simulink model "main_RI_LIEKF"  (R2023a)
settings: Solver=FixedStepAuto  StartTime=0.0  StopTime=220  FixedStep=0.01  RelTol=1e-3
InitFcn:
  | initNavigation0612_AOA;
values from neighbouring files (symbols this model uses):
  CF_enable = 0    [initNavigation.m]
  dt = 0.01    [initNavigation.m]
  dtDelay = -0.03    [initNavigation.m]
  g0 = 9.795    [initNavigation.m]
  gam0_rad = 0/57.3    (= 0)    [initNavigation.m]
  H_sensor_type = 0    [initNavigation.m]
  KF_enable = 1    [initNavigation.m]
  P0 = diag([1*ones(3,1);0.01*ones(3,1);0.1*ones(3,1);0.001*ones(3,1);0.00001*ones(3,1)])    [initNavigation.m]
  P0_RIEKF = diag([1*ones(3,1);0.01*ones(3,1);0.1*ones(3,1);0.001*ones(3,1);0.00001*ones(3,1);      0.01*ones(3,1);[0;2;2]/57.3;[0.1;0.1;0.1]])^2    [initNavigation.m]
  pd0 = 0    [initNavigation.m]
  pe0 = 0    [initNavigation.m]
  phi0_rad = 0/57.3    (= 0)    [initNavigation.m]
  pn0 = 0    [initNavigation.m]
  psi = -178    [initNavigation.m]
  psi0_rad = 0/57.3    (= 0)    [initNavigation.m]
  state_dim = 24    [initNavigation.m]
  Time = 0:0.01:(size(traindata.AttackAngle,1) - 1)*0.01    [NNLiftCoefficientFit.m]
  vd0 = 0    [initNavigation.m]
  ve0 = 0    [initNavigation.m]
  vn0 = 0    [initNavigation.m]
undefined symbols (not defined in the file or in its folder): DiscIntNeverNeededParam, Discrete, INS_CONST, INS_EXPORT, INS_PARAM, magnitude, p, param, pInitialization, sys
libraries: simulink x69, simulink_extras x64, dspstat3 x56, sharedtransform x49, ctrlSharedLib x36, sharedTrackingLibrary x17, FMT_Model_Lib x13, matrix_library x12, deeplib x4, dspsolvers x4, vrlib x4, aerolibconvert2 x1
(part 22 of 22)

== matlab function main_RI_LIEKF/State estimation/bak1/Error State Kalman Filter/Simulink Function - GPS Measurements1/MATLAB Function1 ==
  data: H output; Cbn input; dt input
function H = calH(Cbn, dt)
    

    H = zeros(3,18);
    % 

    H(1:3,4:6) = eye(3);
    H(1:3,16:18) = -Cbn * dt;
end

== matlab function main_RI_LIEKF/State estimation/bak1/Error State Kalman Filter/Simulink Function - State Transition/Cal Phi/MATLAB Function1 ==
  data: vn input; Phi output; pn input; Rbn input; dt input
function Phi = fcn(vn,pn, Rbn,dt)
    
    %{
    F.block(0, 0, 3, 3) = exp_so3(-w_hat * dt);
        F.block(0, 9, 3, 3).noalias() = -exp_so3(-w_hat * dt) * Jr_so3(-w_hat * dt) * dt;
        F.block(9, 9, 3, 3).setIdentity();
        F.block(6, 0, 3, 3).noalias() = -R_Gtoi.transpose() * skew_x(a_hat * dt);
        F.block(6, 6, 3, 3).setIdentity();
        F.block(6, 12, 3, 3) = -R_Gtoi.transpose() * dt;
        F.block(12, 12, 3, 3).setIdentity();
        F.block(3, 0, 3, 3).noalias() = -0.5 * R_Gtoi.transpose() * skew_x(a_hat * dt * dt);
        F.block(3, 6, 3, 3) = Eigen::Matrix3d::Identity() * dt;
        F.block(3, 12, 3, 3) = -0.5 * R_Gtoi.transpose() * dt * dt;
        F.block(3, 3, 3, 3).setIdentity();
        Eigen::Matrix<double, 15, 12> G = Eigen::Matrix<double, 15, 12>::Zero();
    %}
    %
    %
    %F = [0_33         0_33  0_33   -Rbn          0_33]
    %    [skew(gn)     0_33  0_33  -skew(vn)Rbn   -Rbn]
    %    [0.5*skew(gn) I_33  0_33  -skew(pn)Rbn   -Rbn]
    %    [         0_69                  I66          ]
    Phi = zeros(15,15);
    g0 = 9.79;
    gn = [0;0;-g0];
    F  = zeros(15,15);
    F(1:3,10:12) = -Rbn;
    F(4:6,1:3)   = skewMat(gn);
    F(4:6,10:12) = -skewMat(vn)*Rbn;
    F(4:6,13:15) = -Rbn;
    F(7:9,4:6)   = eye(3);
    F(7:9,1:3)   = 0.5*skewMat(gn);
    F(7:9,10:12) = -skewMat(pn)*Rbn;
    F(7:9,13:15) = -Rbn;
    %F(10:15,10:15) = eye(6);
    Phi = eye(15) + F * dt;

end

== matlab function main_RI_LIEKF/State estimation/bak1/Error State Kalman Filter/Simulink Function - State Transition/MATLAB Function ==
  data: Rbn input; G output; vn input; pn input; dt input
function G = fcn(Rbn, vn,pn, dt)
    % G.block(0, 0, 3, 3) = -exp_so3(-w_hat * dt) * Jr_so3(-w_hat * dt) * dt;
    %    G.block(6, 3, 3, 3) = -R_Gtoi.transpose() * dt;
    %    G.block(3, 3, 3, 3) = -0.5 * R_Gtoi.transpose() * dt * dt;
    %    G.block(9, 6, 3, 3).setIdentity();
    %    G.block(12, 9, 3, 3).setIdentity();

    G = zeros(15,12);
    % G(1:3,1:3) = -  Rbn * dt;
    % G(4:6,1:3) = -skewMat(vn)*Rbn* dt;
    % G(4:6,4:6) =  - Rbn;
    % G(7:9,1:3) = -skewMat(pn)*Rbn * dt;
    % G(7:9,4:6) =  - Rbn;
    % G(10:12,7:9) = eye(3)*dt;
    % G(13:15,10:12) = eye(3)*dt;
    G(1:3,1:3) = -  Rbn;
    G(4:6,1:3) = -skewMat(vn)*Rbn;
    G(4:6,4:6) =  - Rbn;
    G(7:9,1:3) = -skewMat(pn)*Rbn;
    G(7:9,4:6) =  - Rbn;
    G(10:12,7:9) = eye(3);
    G(13:15,10:12) = eye(3);
    G = G*double(dt);
end

== matlab function main_RI_LIEKF/State estimation/15dim KF1/Error State Kalman Filter/Cal Phi/MATLAB Function1 ==
  data: axyz input; Phi output; Cnb input; wxyz input; dt input
function Phi = fcn(axyz, Cnb, wxyz,dt)
    
    %{
    F.block(0, 0, 3, 3) = exp_so3(-w_hat * dt);
        F.block(0, 9, 3, 3).noalias() = -exp_so3(-w_hat * dt) * Jr_so3(-w_hat * dt) * dt;
        F.block(9, 9, 3, 3).setIdentity();
        F.block(6, 0, 3, 3).noalias() = -R_Gtoi.transpose() * skew_x(a_hat * dt);
        F.block(6, 6, 3, 3).setIdentity();
        F.block(6, 12, 3, 3) = -R_Gtoi.transpose() * dt;
        F.block(12, 12, 3, 3).setIdentity();
        F.block(3, 0, 3, 3).noalias() = -0.5 * R_Gtoi.transpose() * skew_x(a_hat * dt * dt);
        F.block(3, 6, 3, 3) = Eigen::Matrix3d::Identity() * dt;
        F.block(3, 12, 3, 3) = -0.5 * R_Gtoi.transpose() * dt * dt;
        F.block(3, 3, 3, 3).setIdentity();
        Eigen::Matrix<double, 15, 12> G = Eigen::Matrix<double, 15, 12>::Zero();
    %}
    Phi = zeros(15,15);
    % 
    Phi(1:3,1:3) = eye(3);      %P-P
    Phi(1:3,4:6) = dt * eye(3); %P-V
    Phi(1:3,7:9) = -0.5*Cnb'*skewMat(axyz * dt * dt); %P-the
    % 
    Phi(4:6,4:6) = eye(3);
    Phi(4:6,7:9) = -Cnb' * skewMat(axyz * dt);
    Phi(4:6,10:12) = -Cnb'*dt ;
    % 
    Phi(7:9,7:9) = exp_so3(-wxyz * dt);     %the-the
    Phi(7:9,13:15) = -exp_so3(-wxyz * dt) * Jl_so3(wxyz * dt) * dt; %the-bias g
    % 
    Phi(10:12,10:12) = eye(3);
    % % 
    Phi(13:15,13:15) = eye(3);
    % 
    Phi(1:3,10:12) = - 0.5*Cnb' * dt * dt;

end

== matlab function main_RI_LIEKF/State estimation/ER EKF/INS propogation/Init_PVQ/Horizontal_attitude2/Hem2JPL1 ==
  data: q input; y output
function y = fcn(q)

y = [q(2:4);q(1)];

== matlab function main_RI_LIEKF/State estimation/ER EKF/INS propogation/Init_PVQ/Horizontal_attitude2/Hem2JPL2 ==
  data: q input; y output
function y = fcn(q)

y = [q(2:4);q(1)];

== matlab function main_RI_LIEKF/State estimation/RI EKF/INS propogation/AOA//SA//Vwind update/Subsystem/MATLAB Function3 ==
  data: axyz input; Cy output; TAS input; alpha input; beta input
function Cy = fcn(axyz, TAS,alpha,beta)
ax = axyz(1);
ay = axyz(2);
az = axyz(3);

mess = 6.9;
g = 9.79;
rou = 1.225;
a = 1.4;
b = 0.36;
S = a*b;

q = 0.5 * rou * TAS^2;
ays = -ax .* cos(alpha).*sin(beta) + ay .* cos(beta) - az .* sin(alpha).* sin(beta);
% azs = -ax * sin(alpha) + az * cos(alpha);
Cy = mess * ays / (q * S);
end

== matlab function main_RI_LIEKF/State estimation/RI EKF/INS propogation/AOA//SA//Vwind update/Subsystem/LSTM predict/MATLAB Function5 ==
  data: X input; X_nYPred output
function X_nYPred = LSTMnet(X)
    sig_X = [0.1167;0.1277;0.0579];
    sig_Y = 0.0451;
    mu_X = [0.0587;0.5185;-0.0515];
    mu_Y = 0.1011;
    X_norm = (X - mu_X) ./ sig_X;
    persistent X_nYPredorm_store;
    if isempty(X_nYPredorm_store)
        X_nYPredorm_store = zeros(1000,3);
    end

    X_nYPredorm_store = [X_nYPredorm_store(2:end,:);X_norm'];
    %[~,YPred_seq] = predictAndUpdateState(net.net,X_nYPredorm_store);
     X_nYPred = single(X_nYPredorm_store);
    % YPred_seq = predict(net.net,X_nYPredorm_store');
    % YPred_test = YPred_seq(end);
    % YPred_test = double(YPred_test* sig_Y + mu_Y)*57.3;

end

== matlab function main_RI_LIEKF/State estimation/ER EKF/Error State Kalman Filter/Simulink Function - State Transition/MATLAB Function ==
  data: Cnb input; G output; wxyz input; dt input
function G = fcn(Cnb, wxyz, dt)
    % G.block(0, 0, 3, 3) = -exp_so3(-w_hat * dt) * Jr_so3(-w_hat * dt) * dt;
    %    G.block(6, 3, 3, 3) = -R_Gtoi.transpose() * dt;
    %    G.block(3, 3, 3, 3) = -0.5 * R_Gtoi.transpose() * dt * dt;
    %    G.block(9, 6, 3, 3).setIdentity();
    %    G.block(12, 9, 3, 3).setIdentity();
    
    G = zeros(15,12);
    G(7:9,4:6) = -exp_so3(-wxyz * dt) * Jr_so3(- wxyz * dt) * dt;
    G(1:3,1:3) = -0.5 * Cnb' * dt * dt;
    G(4:6,1:3) = -Cnb' * dt;
    G(10:12,7:9) = eye(3);
    G(13:15,10:12) = eye(3);
    
%     G(16:18,13:15) = eye(3);
%     G(16:18,1:3) = -eye(3);
end

== matlab function main_RI_LIEKF/State estimation/RI EKF/INS propogation/AOA//SA//Vwind update/Subsystem/LSTM predict/MATLAB Function6 ==
  data: YPred_test input; YPred_test_out output
function YPred_test_out = LSTMnet(YPred_test)
    sig_X = [0.1167;0.1277;0.0579];
    sig_Y = 0.0451;
    mu_X = [0.0587;0.5185;-0.0515];
    mu_Y = 0.1011;
    YPred_test_out = YPred_test(end);
    YPred_test_out = single(YPred_test_out* sig_Y + mu_Y)*57.3;

end

== matlab function main_RI_LIEKF/State estimation/15dim KF1/Error State Kalman Filter/Cal Q/MATLAB Function1 ==
  data: Qd output; Cnb input; wxyz input; dt input
function Qd = fcn(Cnb, wxyz, dt)
    % G.block(0, 0, 3, 3) = -exp_so3(-w_hat * dt) * Jr_so3(-w_hat * dt) * dt;
    %    G.block(6, 3, 3, 3) = -R_Gtoi.transpose() * dt;
    %    G.block(3, 3, 3, 3) = -0.5 * R_Gtoi.transpose() * dt * dt;
    %    G.block(9, 6, 3, 3).setIdentity();
    %    G.block(12, 9, 3, 3).setIdentity();
    
    G = zeros(15,12);
    G(7:9,4:6) = -exp_so3(-wxyz * dt) * Jl_so3(wxyz * dt) * dt;
    G(1:3,1:3) = -0.5 * Cnb' * dt * dt;
    G(4:6,1:3) = -Cnb' * dt;
    G(10:12,7:9) = eye(3);
    G(13:15,10:12) = eye(3);
     
    Q = zeros(12,12);
%     noises_sigma_a_2 = 2.0000e-4^2;
%     noises_sigma_w_2 = 1.6968e-4^2;
%     noises_sigma_ab_2 = 3.0000e-4^2;
%     noises_sigma_wb_2 = 1.9393e-5^2;
    noises_sigma_a_2 = 0.0001^2;
    noises_sigma_w_2 = 0.0025^2;
    noises_sigma_ab_2 = 3.0000e-5^2;
    noises_sigma_wb_2 = 0.0002^2;
    Q = diag([noises_sigma_a_2 / dt * ones(3,1); ...
                noises_sigma_w_2 / dt * ones(3,1); ...
                noises_sigma_ab_2 * dt * ones(3,1); ...
                noises_sigma_wb_2 * dt * ones(3,1);]);
    
    Qd = zeros(15,15);
    Qd = G * Q * G';
    Qd = 0.5 * (Qd + Qd');
end

== matlab function main_RI_LIEKF/State estimation/15dim KF1/Error State Kalman Filter/GNSS//INS Kalman Filter1/CalculatePL/Discrete-Time KF - Calculate PLMZ ==
  settings: updateMethod=DISCRETE  sampleTime=pInitialization.Ts
  data: A input; L output; M output; Z output; C input; Q input; R input; N input; P input; PNew output; isEnabled input
function [L,M,Z,PNew] = ctrlKalmanFilterDTCalculatePL_0115(A,C,Q,R,N,P,isEnabled)
% ctrlKalmanFilterDTCalculatePL Calculate the Kalman gain L for current
% time step and P for the next time step (PNew) for discrete-time Kalman
% filtering with time-varying system matrices.
%
%   Inputs:
%     A, C, Q, R, N, P - System and noise covariance matrices. See kalman()
%     isEnabled        - Is measurement update being done at this time
%                        step?
%
%   Outputs:
%      L    - Kalman gain to get x[k+1|k] from x[k|k-1] and y[k]
%      M    - Kalman gain to get x[k|k] from x[k|k-1] and y[k]
%      Z    - State estimation covariance of x[k|k]
%      PNew - P[k+1], state estimation error covariance for the next time
%             step

%   Copyright 2014-2019 The MathWorks, Inc.

%#codegen
if isEnabled
    % Do measurement update
    yCov = C*P*C.'+R;
    L = (A*P*C.'+N) / yCov;
    M = P*C.' / yCov;
    
    Abar = eye(size(A,1),'like', A) - M*C;
    Z = Abar*P*Abar.' + M*R*M.';
    
    NRinv = N/R;
    Abar = A - NRinv*C;
    PNew = Abar*Z*Abar.' + Q - NRinv*N.';
else
    % No measurement update
    L = zeros(size(A,1),size(C,1),'like',A);
    M = L;
    Z = P;
    PNew = A*P*A.' + Q;
end
end

== matlab function main_RI_LIEKF/State estimation/0609bk/Error State Kalman Filter/Extended Kalman Filter1/Correct1/IGG_check/MATLAB Function ==
  data: err input; w output; k0 input; k1 input; zk0 input; zk1 input
function w = fcn(err,k0,k1,zk0,zk1)
    err = abs(err);  w = err;
    for k=1:2
        if err(k)<=k0,    w(k)=1;
        elseif err(k)>k1, w(k)=0;
        else,             w(k)=k0/err(k);  
        end
    end
        if err(3)<=zk0,    w(3)=1;
        elseif err(3)>zk1, w(3)=0;
        else,             w(3)=zk0/err(3);  
        end
end

== matlab function main_RI_LIEKF/State estimation/15dim KF1/Error State Kalman Filter/GNSS//INS Kalman Filter1/CovarianceOutputConfigurator/decideOutput/SqrtUsedFcn ==
  data: u input; P output; isSqrtUsed input
function P = outputCovariance(u,isSqrtUsed)
   
   % Determine if the Square-Root algorithm was used
   if isSqrtUsed
      P = u*u.';
   else
      P = u;
   end   
end

== matlab function main_RI_LIEKF/State estimation/15dim KF1/Error State Kalman Filter/MATLAB Function ==
  data: u input; dp output; dv output; dtheta output; da output; dg output
function [dp,dv,dtheta,da,dg] = fcn(u)
    dp = u(1:3);
    dv = u(4:6);
    dtheta = u(7:9);
    da = u(10:12);
    dg = u(13:15);
end
